simulink model "Traffic_Signals"  (R2022a)
settings: Solver=VariableStepAuto  StartTime=0.0  StopTime=200  RelTol=1e-3
settings Model: Creator=Rohan More  LastModifiedBy=Rohan More

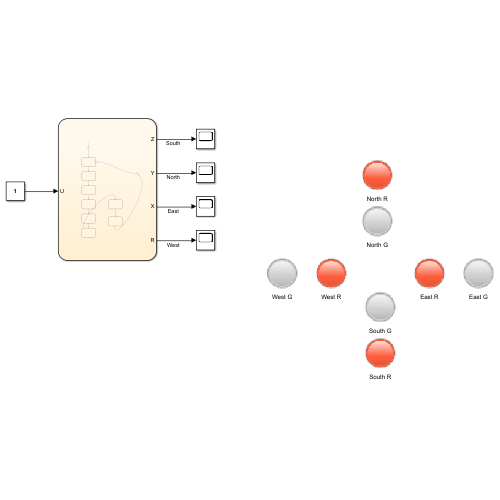
[thumbnail: Simulink's stored preview of the top-level diagram]
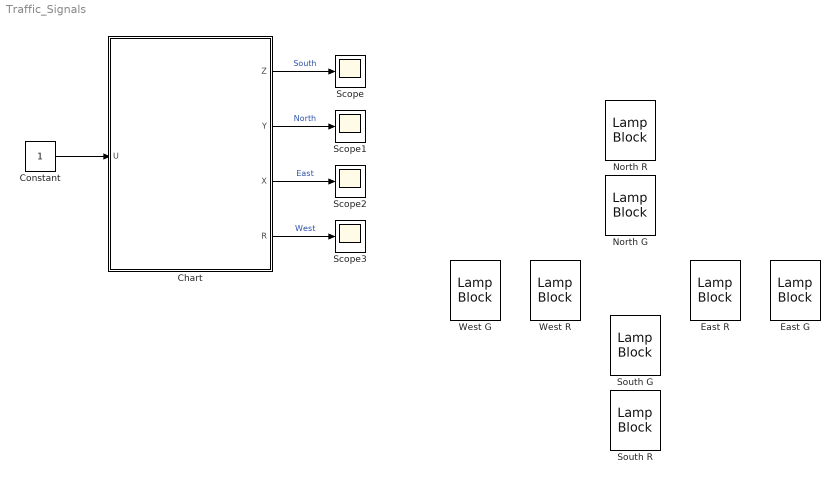
== system Traffic_Signals ==
  Chart : Stateflow chart  TreatAsAtomicUnit=on
  Constant : Constant
  East G : LampBlock  LabelPosition=Hide
  East R : LampBlock  LabelPosition=Hide
  North G : LampBlock  LabelPosition=Hide
  North R : LampBlock  LabelPosition=Hide
  Scope{,1..3} (4 alike) : Scope
  South G : LampBlock  LabelPosition=Hide
  South R : LampBlock  LabelPosition=Hide
  West G : LampBlock  LabelPosition=Hide
  West R : LampBlock  LabelPosition=Hide
  wires:
  Chart/1(Z) -> Scope/1  "South"
  Chart/2(Y) -> Scope1/1  "North"
  Chart/3(X) -> Scope2/1  "East"
  Chart/4(R) -> Scope3/1  "West"
  Constant/1 -> Chart/1(U)

== stateflow chart Traffic_Signals/Chart ==
  state N1
    entry:Y=0
    exit:Y=1
  state N2
    entry:Y=1,Z=1
    exit:Y=0,Z=0
  state E1
    entry:X=0
    exit:X=1
  state E2
    entry:X=1,R=1
    exit:X=0,R=0
  state W1
    entry:R=0
    exit:R=1
  state S1
    entry:Z=0
    exit:Z=1
  state W2
    entry:R=1,X=1
    exit:R=0,X=0
  state S2
    entry:Z=1,Y=1
    exit:Z=0,Y=0
  (default) -> (junction 33)
  (junction 33) -> N1
  (junction 20) -> N1
  N1 -> N2 : after(20,sec)[U==1]
  W2 -> (junction 20) : after(60,sec)
  N2 -> E1 : after(40,sec)
  S2 -> W1 : after(120,sec)
  E1 -> E2 : after(60,sec)
  E2 -> S1 : after(80,sec)
  W1 -> W2 : after(140,sec)
  S1 -> S2 : after(100,sec)
  data: Z output; Y output; X output; R output; U input
